simulink model "sislinear"  (R2023b)
settings: Solver=VariableStepAuto  StartTime=0.0  StopTime=10.0  RelTol=1e-3
settings Model: Creator=Geovanne  LastModifiedBy=Geovanne

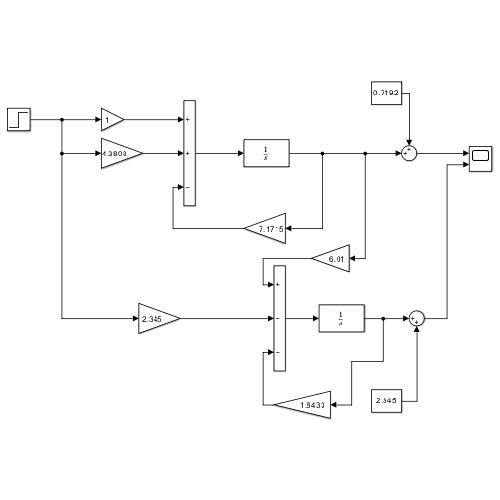
[thumbnail: Simulink's stored preview of the top-level diagram]
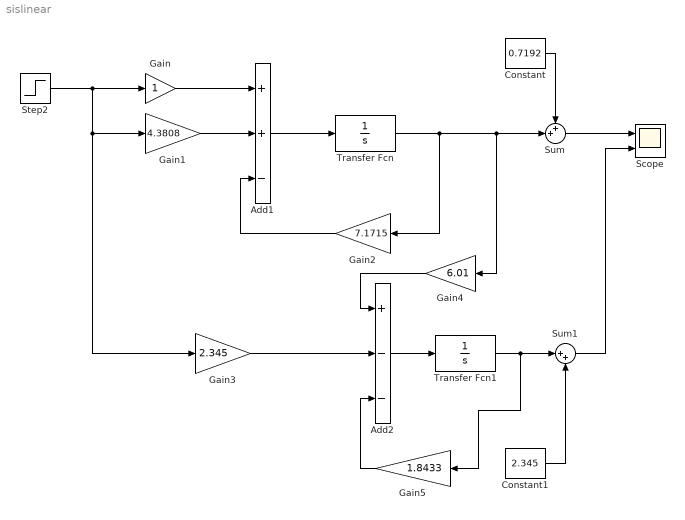
== system sislinear ==
  Add1 : Sum  Inputs=++-
  Add2 : Sum  Inputs=+--
  Constant : Constant  Value=0.7192
  Constant1 : Constant  Value=2.345
  Gain : Gain
  Gain1 : Gain  Gain=4.3808
  Gain2 : Gain  Gain=7.1715
  Gain3 : Gain  Gain=2.345
  Gain4 : Gain  Gain=6.01
  Gain5 : Gain  Gain=1.8433
  Scope : Scope  NumInputPorts=2
  Step2 : Step  After=0.1  SampleTime=0
  Sum : Sum  Inputs=++|
  Sum1 : Sum  Inputs=|++
  Transfer Fcn : TransferFcn  Denominator=[1 0]
  Transfer Fcn1 : TransferFcn  Denominator=[1 0]
  wires:
  Step2/1 -> Gain3/1, Gain1/1, Gain/1
  Gain/1 -> Add1/1
  Gain1/1 -> Add1/2
  Add1/1 -> Transfer Fcn/1
  Transfer Fcn/1 -> Gain4/1, Sum/2, Gain2/1
  Sum/1 -> Scope/1
  Gain2/1 -> Add1/3
  Constant/1 -> Sum/1
  Gain4/1 -> Add2/1
  Gain3/1 -> Add2/2
  Add2/1 -> Transfer Fcn1/1
  Sum1/1 -> Scope/2
  Transfer Fcn1/1 -> Gain5/1, Sum1/1
  Constant1/1 -> Sum1/2
  Gain5/1 -> Add2/3
